simulink model "NoSuspensionSSC"  (R2026b)
settings: Solver=VariableStepAuto
settings Model: Creator=The MathWorks, Inc.  LastModifiedBy=The MathWorks, Inc.
settings DebuggingCC: SubsystemReferenceDiagnosticForUnitTest=warning

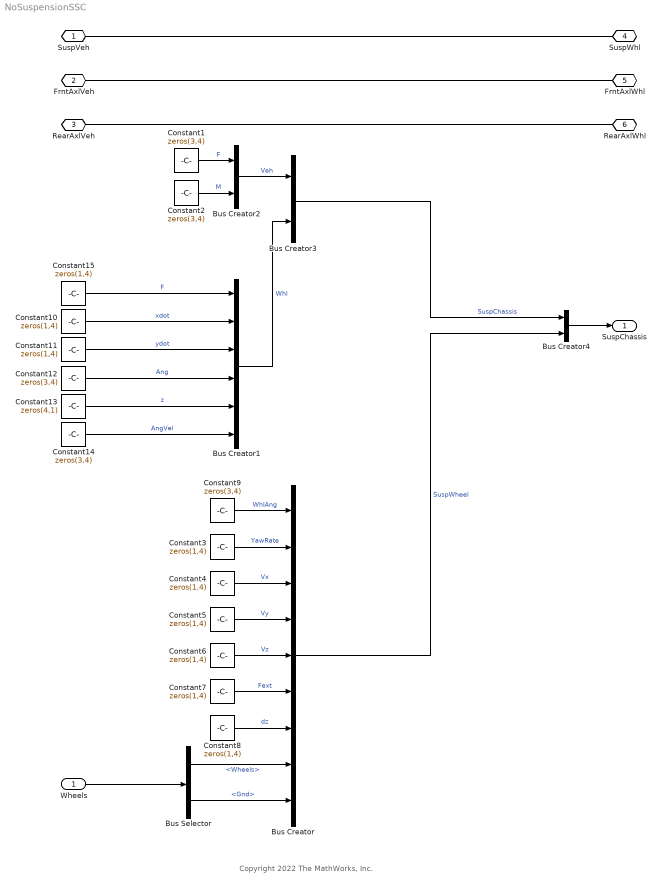
== system NoSuspensionSSC ==
  note: Copyright 2022 The MathWorks, Inc.
  Wheels : Inport
  Bus Creator : BusCreator  Inputs=9
  Bus Creator1 : BusCreator  Inputs=6
  Bus Creator2 : BusCreator  Inputs=2
  Bus Creator3 : BusCreator  Inputs=2
  Bus Creator4 : BusCreator  Inputs=2
  Bus Selector : BusSelector  OutputSignals=Wheels,Gnd
  Constant{1..2,9,12,14} (5 alike) : Constant  Value=zeros(3,4)  SampleTime=-1
  Constant{3..8,10..11,15} (9 alike) : Constant  Value=zeros(1,4)  SampleTime=-1
  Constant13 : Constant  Value=zeros(4,1)  SampleTime=-1
  SuspVeh : PMIOPort  Side=Left
  FrntAxlVeh : PMIOPort  Port=2  Side=Left
  RearAxlVeh : PMIOPort  Port=3  Side=Left
  SuspWhl : PMIOPort  Port=4  Side=Right
  FrntAxlWhl : PMIOPort  Port=5  Side=Right
  RearAxlWhl : PMIOPort  Port=6  Side=Right
  SuspChassis : Outport
  wires:
  Bus Creator/1 -> Bus Creator4/2  "SuspWheel"
  Constant10/1 -> Bus Creator1/2  "xdot"
  Bus Creator3/1 -> Bus Creator4/1  "SuspChassis"
  Bus Creator4/1 -> SuspChassis/1
  Bus Creator1/1 -> Bus Creator3/2  "Whl"
  Constant11/1 -> Bus Creator1/3  "ydot"
  Constant12/1 -> Bus Creator1/4  "Ang"
  Constant13/1 -> Bus Creator1/5  "z"
  Constant14/1 -> Bus Creator1/6  "AngVel"
  Constant15/1 -> Bus Creator1/1  "F"
  Constant5/1 -> Bus Creator/4  "Vy"
  Bus Selector/1 -> Bus Creator/8  "<Wheels>"
  Constant6/1 -> Bus Creator/5  "Vz"
  Constant9/1 -> Bus Creator/1  "WhlAng"
  Constant4/1 -> Bus Creator/3  "Vx"
  Bus Selector/2 -> Bus Creator/9  "<Gnd>"
  Constant8/1 -> Bus Creator/7  "dz"
  Constant3/1 -> Bus Creator/2  "YawRate"
  Constant7/1 -> Bus Creator/6  "Fext"
  Wheels/1 -> Bus Selector/1
  Constant2/1 -> Bus Creator2/2  "M"
  Bus Creator2/1 -> Bus Creator3/1  "Veh"
  Constant1/1 -> Bus Creator2/1  "F"
  connections:
  RearAxlVeh/RConn1 -- RearAxlWhl/RConn1
  SuspVeh/RConn1 -- SuspWhl/RConn1
  FrntAxlVeh/RConn1 -- FrntAxlWhl/RConn1
